simulink subsystem "Motores"  (R2023b)
settings: Solver=VariableStepAuto  StartTime=0.0  StopTime=10.0  RelTol=1e-3
libraries: arduinolib x4
settings Model: Creator=Enrique  LastModifiedBy=Enrique

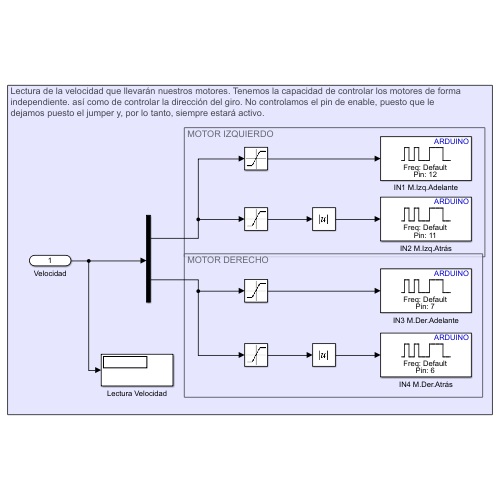
[thumbnail: Simulink's stored preview of the top-level diagram]
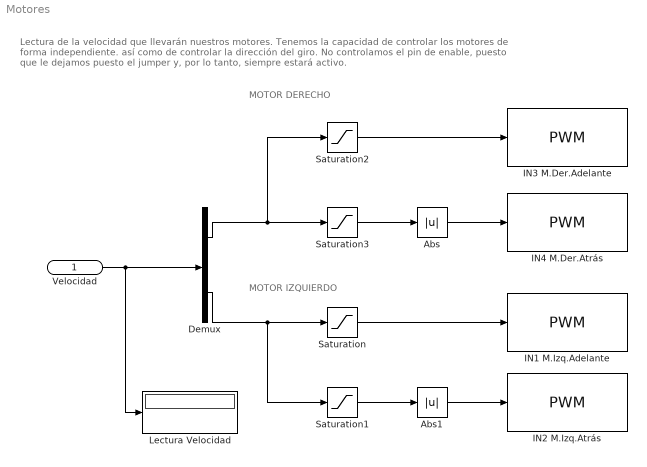
== system Motores ==
  note: MOTOR DERECHO
  note: MOTOR IZQUIERDO
  note: Lectura de la velocidad que llevarán nuestros motores. Tenemos la capacidad de controlar los motores de forma
      | independiente. así como de controlar la dirección del giro. No controlamos el pin de enable, puesto que le
      | dejamos puesto el jumper y, por lo tanto, siempre estará activo.
  Velocidad : Inport
  Abs : Abs  SaturateOnIntegerOverflow=off
  Abs1 : Abs  SaturateOnIntegerOverflow=off
  Demux : Demux  Outputs=2
  IN1 M.Izq.Adelante : arduinolib/PWM  pinNumber=12  frequencyType=Default  desiredFrequency=490.2  achievableFrequency=490.2
  IN2 M.Izq.Atrás : arduinolib/PWM  pinNumber=11  frequencyType=Default  desiredFrequency=490.2  achievableFrequency=490.2
  IN3 M.Der.Adelante : arduinolib/PWM  pinNumber=6  frequencyType=Default  desiredFrequency=490.2  achievableFrequency=490.2
  IN4 M.Der.Atrás : arduinolib/PWM  pinNumber=7  frequencyType=Default  desiredFrequency=490.2  achievableFrequency=490.2
  Lectura Velocidad : Display
  Saturation : Saturate  UpperLimit=255  LowerLimit=0
  Saturation1 : Saturate  UpperLimit=0  LowerLimit=-255
  Saturation2 : Saturate  UpperLimit=255  LowerLimit=0
  Saturation3 : Saturate  UpperLimit=0  LowerLimit=-255
  wires:
  Velocidad/1 -> Demux/1, Lectura Velocidad/1
  Saturation1/1 -> Abs1/1
  Saturation3/1 -> Abs/1
  Saturation2/1 -> IN3 M.Der.Adelante/1
  Abs/1 -> IN4 M.Der.Atrás/1
  Saturation/1 -> IN1 M.Izq.Adelante/1
  Abs1/1 -> IN2 M.Izq.Atrás/1
  Demux/1 -> Saturation3/1, Saturation2/1
  Demux/2 -> Saturation/1, Saturation1/1
